simulink model "Observateur_step2_Retour_etat"  (R2019a)
settings: Solver=VariableStepAuto  StartTime=0.0  StopTime=2  RelTol=1e-3
undefined symbols (not defined in the file): A, Ao, B, Bo, C, Co, G, Kc, Ko, u0, uf, x0, xo0
settings Model: Creator=Alex  LastModifiedBy=Alex

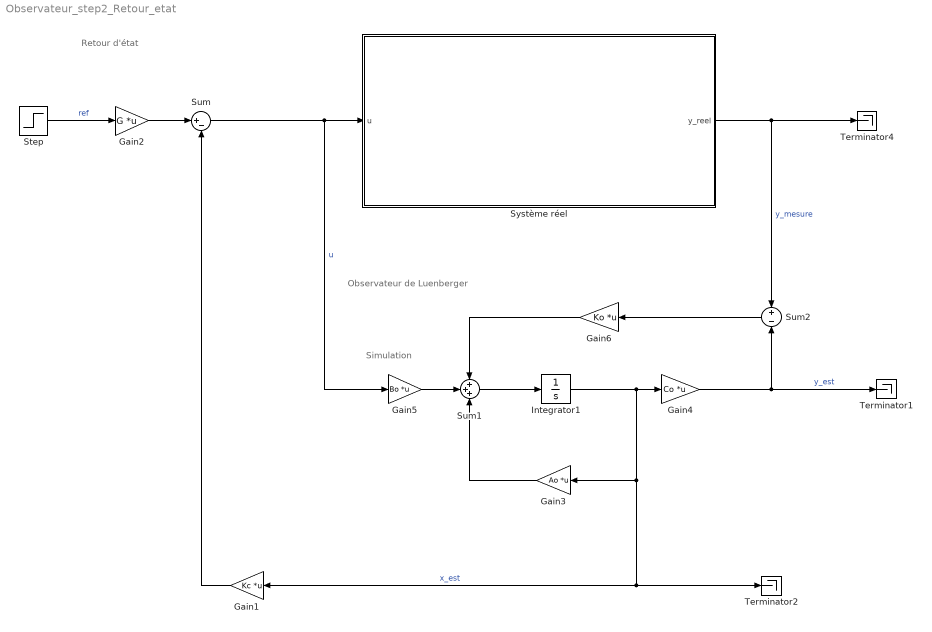
== system Observateur_step2_Retour_etat ==
  note: Retour d'état
  note: Observateur de Luenberger
  note: Simulation
  Gain1 : Gain  Gain=Kc  Multiplication=Matrix(K*u)
  Gain2 : Gain  Gain=G  Multiplication=Matrix(K*u)
  Gain3 : Gain  Gain=Ao  Multiplication=Matrix(K*u)
  Gain4 : Gain  Gain=Co  Multiplication=Matrix(K*u)
  Gain5 : Gain  Gain=Bo  Multiplication=Matrix(K*u)
  Gain6 : Gain  Gain=Ko  Multiplication=Matrix(K*u)
  Integrator1 : Integrator  InitialCondition=xo0
      settings: AttributesFormatString=Conditions intiales %<InitialCondition>
  Step : Step  Before=u0  After=uf  SampleTime=0
  Sum : Sum  Inputs=|+-
  Sum1 : Sum  Inputs=+++
  Sum2 : Sum  Inputs=+-
  Système réel : Subsystem
  Terminator1 : Terminator
  Terminator2 : Terminator
  Terminator4 : Terminator
  wires:
  Système réel/1(y_reel) -> Sum2/1, Terminator4/1  "y_mesure"
  Sum/1 -> Gain5/1, Système réel/1(u)  "u"
  Integrator1/1 -> Terminator2/1, Gain1/1, Gain3/1, Gain4/1  "x_est"
  Sum1/1 -> Integrator1/1
  Gain4/1 -> Terminator1/1, Sum2/2  "y_est"
  Sum2/1 -> Gain6/1
  Gain5/1 -> Sum1/2
  Gain3/1 -> Sum1/3
  Gain6/1 -> Sum1/1
  Step/1 -> Gain2/1  "ref"
  Gain2/1 -> Sum/1
  Gain1/1 -> Sum/2

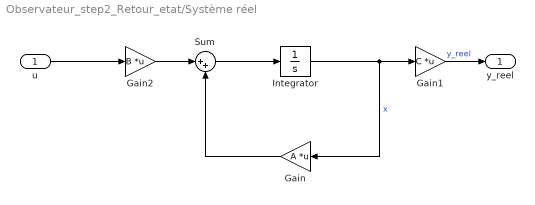
== system Observateur_step2_Retour_etat/Système réel ==
  u : Inport
  Gain : Gain  Gain=A  Multiplication=Matrix(K*u)
  Gain1 : Gain  Gain=C  Multiplication=Matrix(K*u)
  Gain2 : Gain  Gain=B  Multiplication=Matrix(K*u)
  Integrator : Integrator  InitialCondition=x0
      settings: AttributesFormatString=Conditions intiales %<InitialCondition>
  Sum : Sum  Inputs=|++
  y_reel : Outport
  wires:
  Sum/1 -> Integrator/1
  Gain2/1 -> Sum/1
  Integrator/1 -> Gain1/1, Gain/1  "x"
  Gain1/1 -> y_reel/1  "y_reel"
  u/1 -> Gain2/1
  Gain/1 -> Sum/2
